simulink model "Counter"  (R2021b)
settings: Solver=VariableStepAuto  StartTime=0.0  StopTime=10  RelTol=1e-3
undefined symbols (not defined in the file): sigbuilder_block
settings Model: Creator=mohamednasser  LastModifiedBy=mohamednasser

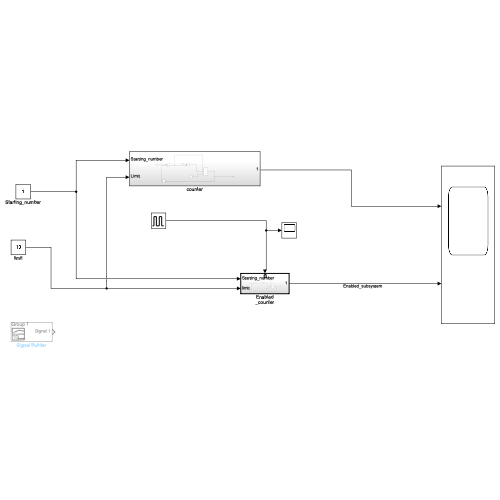
[thumbnail: Simulink's stored preview of the top-level diagram]
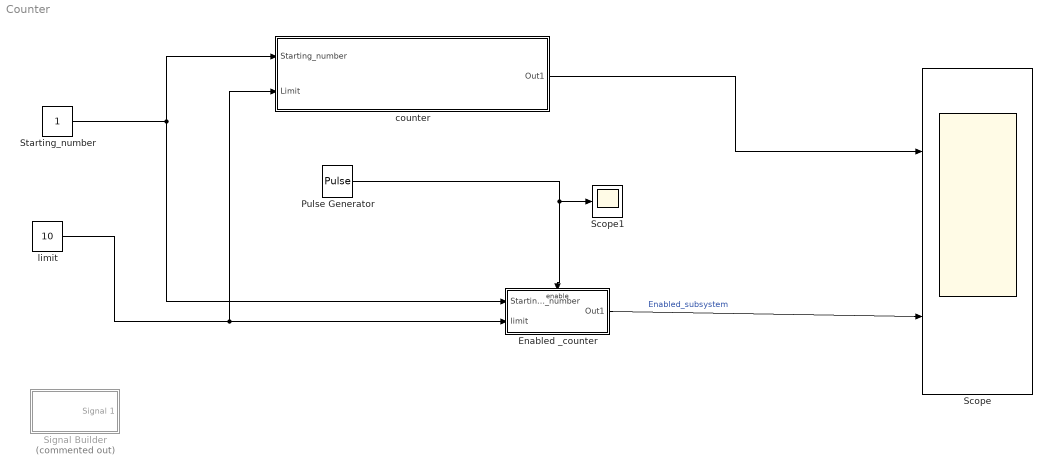
== system Counter ==
  Enabled _counter : Subsystem  TreatAsAtomicUnit=on
  Pulse Generator : DiscretePulseGenerator  PulseType=Time based  Period=0.1  PulseWidth=50
  Scope : Scope  NumInputPorts=2
  Scope1 : Scope
  Signal Builder : Subsystem  Tag=STV Subsys  Commented=on  LoadFcn=sigbuilder_block('load');  StartFcn=sigbuilder_block('start');  StopFcn=sigbuilder_block('stop');  ClipboardFcn=sigbuilder_block('clipboard');  mask(Sigbuilder block){tuvar=[0:10]}
      mask help: Simulink:masks:SigbuilderBlock_MD
      mask init:
      | if ~strcmp(get_param(bdroot(gcbh),'SimulationStatus'),'stopped') tuvar = sigbuilder_block('maskInit'); end
      settings: CopyFcn=sigbuilder_block('copy');  DeleteFcn=sigbuilder_block('delete');  ModelCloseFcn=sigbuilder_block('modelClose');  PreSaveFcn=sigbuilder_block('preSave');  PauseFcn=sigbuilder_block('pause');  ContinueFcn=sigbuilder_block('continue');  NameChangeFcn=sigbuilder_block('namechange');  OpenFcn=sigbuilder_block('open',[437.6 199.2 550.4 400 ]);  CloseFcn=sigbuilder_block('close');
      mask Display: plot(0, 0, 100, 100,[2, 2, 32, 32, 2], [68, 8, 8, 68, 68],[32, 2], [38, 38], [32, 19, 2],[53, 60, 44], [32, 17, 17, 2],[16, 16, 31, 31]);txt = getActiveGroup(gcbh);text(2, 100, txt,'verticalAlignment', 'top');
  Starting_number : Constant
  counter : Subsystem
  limit : Constant  Value=10
  wires:
  Enabled _counter/1(Out1) -> Scope/2  "Enabled_subsystem"
  Starting_number/1 -> counter/1(Starting_number), Enabled _counter/1(Starting_number)
  counter/1(Out1) -> Scope/1
  Pulse Generator/1 -> Scope1/1, Enabled _counter/Enable
  limit/1 -> counter/2(Limit), Enabled _counter/2(limit)

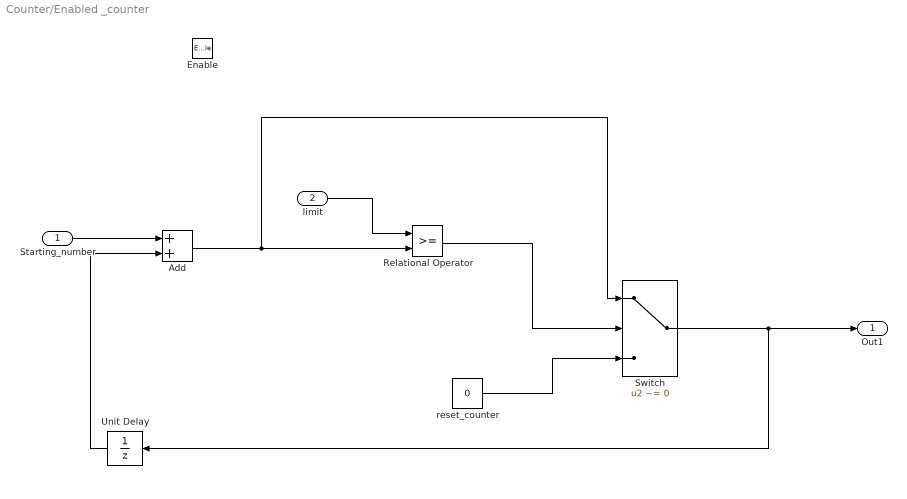
== system Counter/Enabled _counter ==
  Starting_number : Inport
  limit : Inport  Port=2
  Enable : EnablePort
  Add : Sum
  Relational Operator : RelationalOperator  OutDataTypeStr=boolean  RndMeth=Simplest
  Switch : Switch  Criteria=u2 ~= 0
  Unit Delay : UnitDelay  SampleTime=-1  HasFrameUpgradeWarning=on
  reset_counter : Constant  Value=0
  Out1 : Outport
  wires:
  Unit Delay/1 -> Add/2
  Add/1 -> Switch/1, Relational Operator/2
  Switch/1 -> Out1/1, Unit Delay/1
  reset_counter/1 -> Switch/3
  Starting_number/1 -> Add/1
  Relational Operator/1 -> Switch/2
  limit/1 -> Relational Operator/1

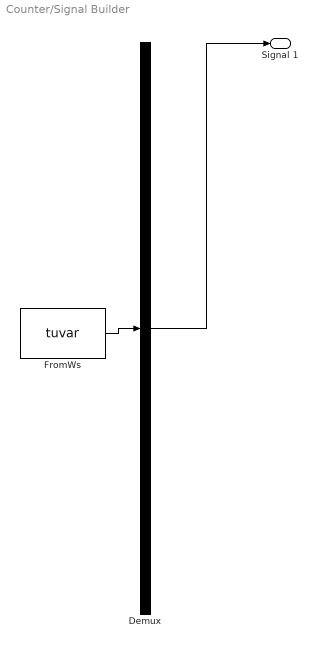
== system Counter/Signal Builder ==
  Demux : Demux  Tag=STV Demux  Outputs=1
      settings: DisplayOption=none
  FromWs : FromWorkspace  Tag=STV FromWs  VariableName=tuvar
      SigBuilderData=|
      | common.afterFinalStr = 'Extrapolate'
      | common.sampleTime = 0
      | dataSet.timeRange = [0 10]
      | dataSet.name = 'Group 1'
      | sbobj.Groups.Name = 'Group 1'
      | sbobj.Groups.Signals.Name = 'Signal 1'
      | sbobj.Groups.Signals.XData = [0 4 6 10]
      | sbobj.Groups.Signals.YData = [1 1 1 1]
  Signal 1 : Outport  Tag=STV Outport
  wires:
  Demux/1 -> Signal 1/1
  FromWs/1 -> Demux/1

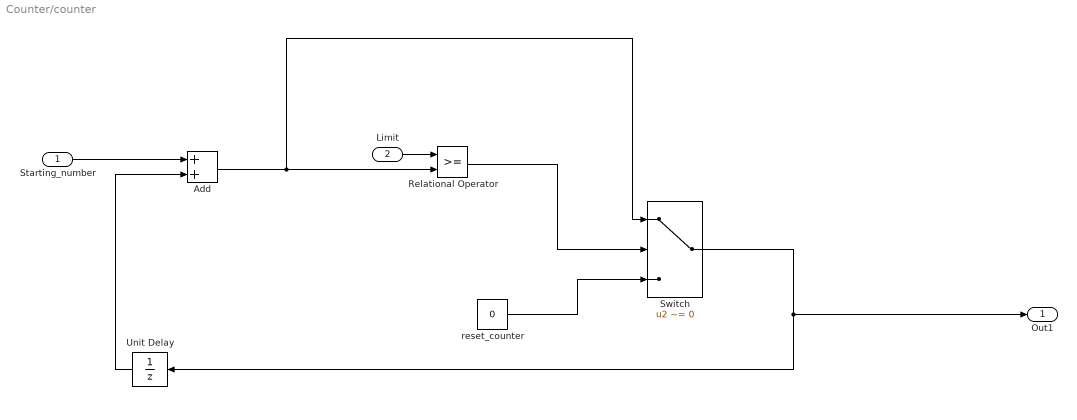
== system Counter/counter ==
  Starting_number : Inport
  Limit : Inport  Port=2
  Add : Sum
  Relational Operator : RelationalOperator  OutDataTypeStr=boolean  RndMeth=Simplest
  Switch : Switch  Criteria=u2 ~= 0
  Unit Delay : UnitDelay  SampleTime=-1  HasFrameUpgradeWarning=on
  reset_counter : Constant  Value=0
  Out1 : Outport
  wires:
  Relational Operator/1 -> Switch/2
  Starting_number/1 -> Add/1
  reset_counter/1 -> Switch/3
  Switch/1 -> Out1/1, Unit Delay/1
  Add/1 -> Switch/1, Relational Operator/2
  Unit Delay/1 -> Add/2
  Limit/1 -> Relational Operator/1
